simulink model "BUCK_BUCKBOOST_R2023b"  (R2023b)
settings: Solver=ode3  StartTime=0.0  StopTime=1  RelTol=1e-3
libraries: spsSeriesRLCBranchLib x56, spsCurrentMeasurementLib x42, spsVoltageMeasurementLib x27, spsMosfetLib x20, spsDiodeLib x18, spsPWMGeneratorDCDCLib x18, spsDCVoltageSourceLib x7, spsControlledVoltageSourceLib x2, spspowerguiLib x1
settings Model: Creator=tharu  LastModifiedBy=tharu
settings RTWCC: GPUComputeCapability=5.0
settings ConfigComp: CovBoundaryAbsTol=1.0e-5

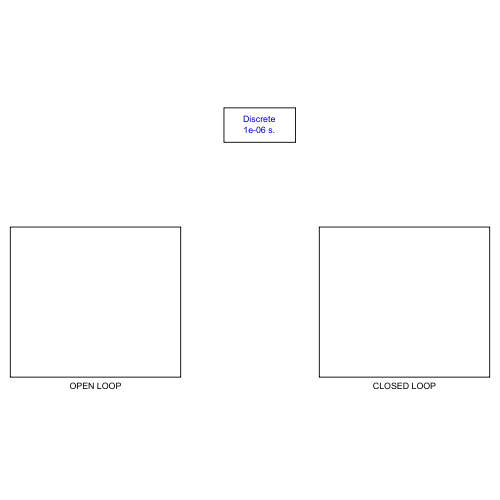
[thumbnail: Simulink's stored preview of the top-level diagram]
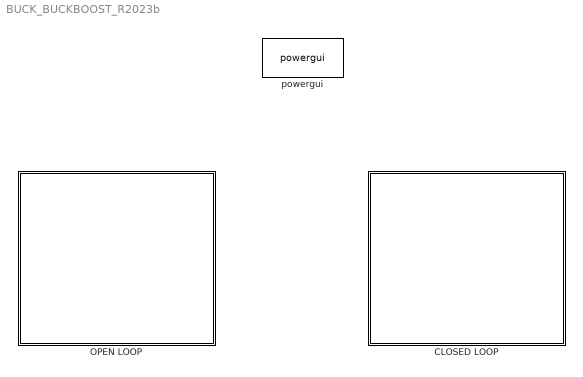
== system BUCK_BUCKBOOST_R2023b ==
  CLOSED LOOP : Subsystem
  OPEN LOOP : Subsystem
  powergui : spspowerguiLib/powergui  Priority=1  SimulationMode=Discrete  SampleTime=1e-6  frequency=60  Iterations=50  frequencyindice=0  Pbase=100e6  ErrMax=1e-4  UnitsV=kV  UnitsW=MW  buscounter=0  FunctionMessages=off  echomessages=off  EnableUseOfTLC=off  CurrentSourceSwitches=off  DisableSnubberDevices=off  DisableRonSwitches=off  DisableVfSwitches=off  DisplayEquations=off  AutomaticDiscreteSolvers=off  SolverType=Tustin/Backward Euler (TBE)  Interpol=off  ExternalGateDelay=off  methode=off  Ts=100  x0status=blocks  SPID=on  SwTol=0  HookPort=off  NonlinearTolerance=1e-4  nMaxIteration=100  ContinueOnMaxIteration=off  RestoreLinks=warning  ResistiveCurrentMeasurement=off  Frange=[0:2:500]  Ylog=off  Xlog=on  ShowGrid=off  save=off  variable=ZData  structure=0  ZoomFFT=off  StartTime=0.0  cycles=1  DisplayStyle=1  fundamental=60  FreqAxis=off  MaxFrequency=1000  frequencyindicesteady=1  RmsSteady=1  display=off

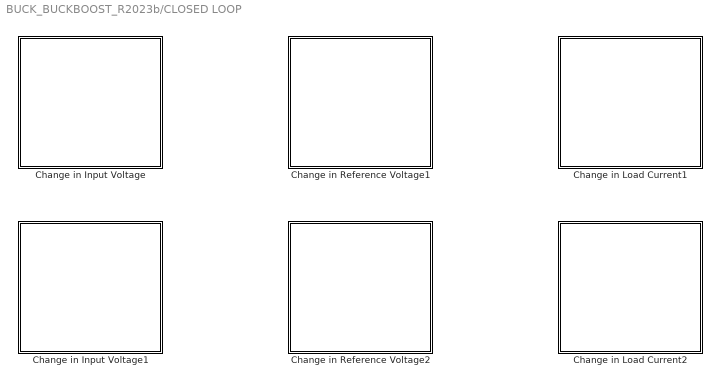
== system BUCK_BUCKBOOST_R2023b/CLOSED LOOP ==
  Change in Input Voltage : Subsystem
  Change in Input Voltage1 : Subsystem
  Change in Load Current1 : Subsystem
  Change in Load Current2 : Subsystem
  Change in Reference Voltage1 : Subsystem
  Change in Reference Voltage2 : Subsystem

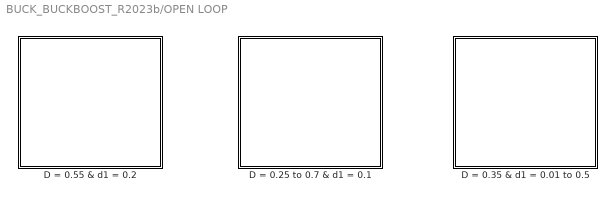
== system BUCK_BUCKBOOST_R2023b/OPEN LOOP ==
  D = 0.25 to 0.7 & d1 = 0.1 : Subsystem
  D = 0.35 & d1 = 0.01 to 0.5 : Subsystem
  D = 0.55 & d1 = 0.2 : Subsystem

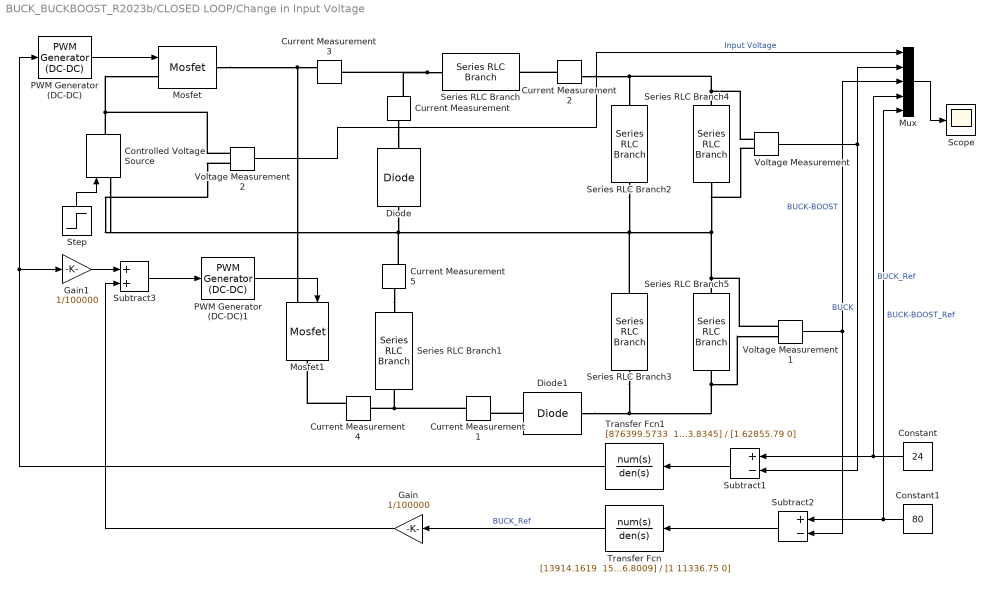
== system BUCK_BUCKBOOST_R2023b/CLOSED LOOP/Change in Input Voltage ==
  Constant : Constant  Value=24
  Constant1 : Constant  Value=80
  Controlled Voltage Source : spsControlledVoltageSourceLib/Controlled Voltage Source  Initialize=on  Source_Type=AC  Amplitude=0  Phase=0  Frequency=0  Measurements=None
  Current Measurement{,1..5} (6 alike) : spsCurrentMeasurementLib/Current Measurement  PhasorSimulation=off  OutputType=Complex  PSBequivalent=0
  Diode : spsDiodeLib/Diode  Ron=0.001  Lon=0  Vf=0.8  IC=0  UseSnubber=0  Rs=500  Cs=250e-9  Measurements=off
  Diode1 : spsDiodeLib/Diode  Ron=0.001  Lon=0  Vf=0.8  IC=0  UseSnubber=0  Rs=500  Cs=250e-9  Measurements=off
  Gain : Gain  Gain=1/100000
  Gain1 : Gain  Gain=1/100000
  Mosfet : spsMosfetLib/Mosfet  Ron=0.1  Lon=0  Rd=0.01  Vfd=0  IC=0  Rs=1e5  Cs=inf  Measurements=off
  Mosfet1 : spsMosfetLib/Mosfet  Ron=0.1  Lon=0  Rd=0.01  Vfd=0  IC=0  Rs=1e5  Cs=inf  Measurements=off
  Mux : Mux  Inputs=5
  PWM Generator (DC-DC) : spsPWMGeneratorDCDCLib/PWM Generator (DC-DC)  Fsw=50000  Ts=0
  PWM Generator (DC-DC)1 : spsPWMGeneratorDCDCLib/PWM Generator (DC-DC)  Fsw=50000  Ts=0
  Scope : Scope
  Series RLC Branch : spsSeriesRLCBranchLib/Series RLC Branch  LConnTagsString=__new0  RConnTagsString=__new0  BranchType=L  Resistance=1  Inductance=2e-3  SetiL0=off  InitialCurrent=0  Capacitance=1e-6  Setx0=off  InitialVoltage=0  Measurements=None
  Series RLC Branch1 : spsSeriesRLCBranchLib/Series RLC Branch  LConnTagsString=__new0  RConnTagsString=__new0  BranchType=L  Resistance=1  Inductance=600e-6  SetiL0=off  InitialCurrent=0  Capacitance=1e-6  Setx0=off  InitialVoltage=0  Measurements=None
  Series RLC Branch2 : spsSeriesRLCBranchLib/Series RLC Branch  LConnTagsString=__new0  RConnTagsString=__new0  BranchType=C  Resistance=1  Inductance=1e-3  SetiL0=off  InitialCurrent=0  Capacitance=100e-6  Setx0=off  InitialVoltage=0  Measurements=None
  Series RLC Branch3 : spsSeriesRLCBranchLib/Series RLC Branch  LConnTagsString=__new0  RConnTagsString=__new0  BranchType=C  Resistance=1  Inductance=1e-3  SetiL0=off  InitialCurrent=0  Capacitance=100e-6  Setx0=off  InitialVoltage=0  Measurements=None
  Series RLC Branch4 : spsSeriesRLCBranchLib/Series RLC Branch  LConnTagsString=__new0  RConnTagsString=__new0  BranchType=R  Resistance=100  Inductance=1e-3  SetiL0=off  InitialCurrent=0  Capacitance=1e-6  Setx0=off  InitialVoltage=0  Measurements=None
  Series RLC Branch5 : spsSeriesRLCBranchLib/Series RLC Branch  LConnTagsString=__new0  RConnTagsString=__new0  BranchType=R  Resistance=100  Inductance=1e-3  SetiL0=off  InitialCurrent=0  Capacitance=1e-6  Setx0=off  InitialVoltage=0  Measurements=None
  Step : Step  Time=0.5  Before=48  After=40  SampleTime=0
  Subtract1 : Sum  Inputs=+-
  Subtract2 : Sum  Inputs=+-
  Subtract3 : Sum
  Transfer Fcn : TransferFcn  Numerator="[13914.1619  15610474.6386 3044445646.8009]"  Denominator=[1 11336.75 0]
  Transfer Fcn1 : TransferFcn  Numerator="[876399.5733  1811059206.4392 399810634503.8345]"  Denominator=[1 62855.79 0]
  Voltage Measurement : spsVoltageMeasurementLib/Voltage Measurement  PhasorSimulation=off  OutputType=Complex  PSBequivalent=0
  Voltage Measurement1 : spsVoltageMeasurementLib/Voltage Measurement  PhasorSimulation=off  OutputType=Complex  PSBequivalent=0
  Voltage Measurement2 : spsVoltageMeasurementLib/Voltage Measurement  PhasorSimulation=off  OutputType=Complex  PSBequivalent=0
  wires:
  PWM Generator (DC-DC)/1 -> Mosfet/1
  Voltage Measurement1/1 -> Subtract2/2, Mux/3  "BUCK-BOOST"
  Voltage Measurement/1 -> Subtract1/2, Mux/2  "BUCK"
  Constant/1 -> Mux/4, Subtract1/1  "BUCK_Ref"
  Constant1/1 -> Subtract2/1, Mux/5  "BUCK-BOOST_Ref"
  Step/1 -> Controlled Voltage Source/1
  Mux/1 -> Scope/1
  Subtract1/1 -> Transfer Fcn1/1
  Voltage Measurement2/1 -> Mux/1  "Input Voltage"
  Subtract2/1 -> Transfer Fcn/1
  Transfer Fcn/1 -> Gain/1  "BUCK_Ref"
  Gain/1 -> Subtract3/2
  Transfer Fcn1/1 -> PWM Generator (DC-DC)/1, Gain1/1
  Gain1/1 -> Subtract3/1
  Subtract3/1 -> PWM Generator (DC-DC)1/1
  PWM Generator (DC-DC)1/1 -> Mosfet1/1
  connections:
  Diode1/LConn1 -- Series RLC Branch3/RConn1 -- Voltage Measurement1/LConn2 -- Series RLC Branch5/RConn1
  Series RLC Branch4/LConn1 -- Voltage Measurement/LConn1 -- Current Measurement2/RConn1 -- Series RLC Branch2/LConn1
  Series RLC Branch5/LConn1 -- Voltage Measurement1/LConn1 -- Voltage Measurement/LConn2 -- Series RLC Branch4/RConn1 -- Controlled Voltage Source/LConn1 -- Voltage Measurement2/LConn2 -- Current Measurement5/RConn1 -- Diode/LConn1 -- Series RLC Branch3/LConn1 -- Series RLC Branch2/RConn1
  Current Measurement1/LConn1 -- Series RLC Branch1/RConn1 -- Current Measurement4/LConn1
  Series RLC Branch/LConn1 -- Current Measurement/RConn1 -- Current Measurement3/LConn1
  Voltage Measurement2/LConn1 -- Controlled Voltage Source/RConn1 -- Mosfet/LConn1
  Diode1/RConn1 -- Current Measurement1/RConn1
  Current Measurement2/LConn1 -- Series RLC Branch/RConn1
  Current Measurement5/LConn1 -- Series RLC Branch1/LConn1
  Mosfet/RConn1 -- Mosfet1/LConn1 -- Current Measurement3/RConn1
  Current Measurement4/RConn1 -- Mosfet1/RConn1
  Current Measurement/LConn1 -- Diode/RConn1

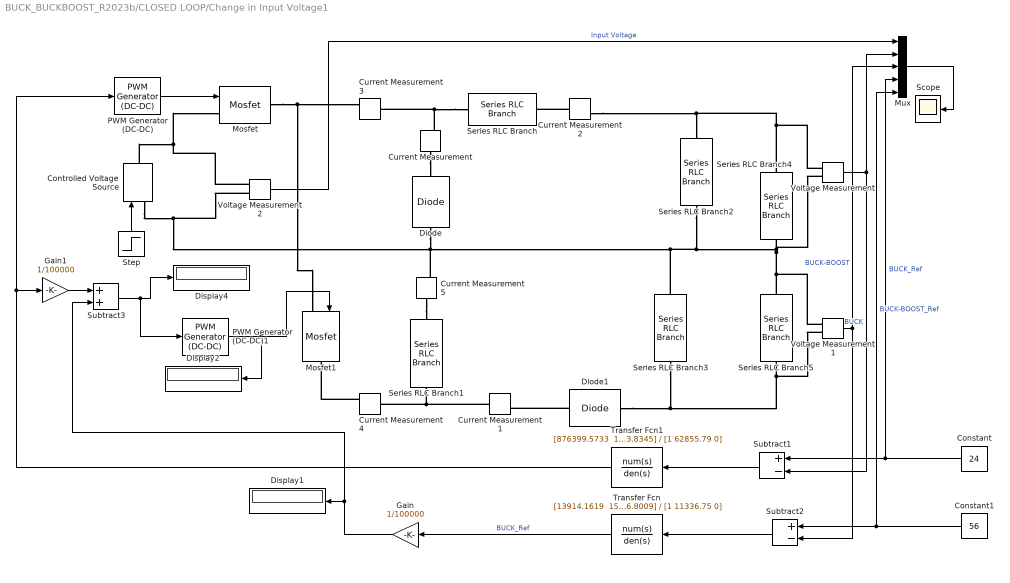
== system BUCK_BUCKBOOST_R2023b/CLOSED LOOP/Change in Input Voltage1 ==
  Constant : Constant  Value=24
  Constant1 : Constant  Value=56
  Controlled Voltage Source : spsControlledVoltageSourceLib/Controlled Voltage Source  Initialize=on  Source_Type=AC  Amplitude=0  Phase=0  Frequency=0  Measurements=None
  Current Measurement{,1..5} (6 alike) : spsCurrentMeasurementLib/Current Measurement  PhasorSimulation=off  OutputType=Complex  PSBequivalent=0
  Diode : spsDiodeLib/Diode  Ron=0.001  Lon=0  Vf=0.8  IC=0  UseSnubber=0  Rs=500  Cs=250e-9  Measurements=off
  Diode1 : spsDiodeLib/Diode  Ron=0.001  Lon=0  Vf=0.8  IC=0  UseSnubber=0  Rs=500  Cs=250e-9  Measurements=off
  Display1 : Display
  Display2 : Display
  Display4 : Display
  Gain : Gain  Gain=1/100000
  Gain1 : Gain  Gain=1/100000
  Mosfet : spsMosfetLib/Mosfet  Ron=0.1  Lon=0  Rd=0.01  Vfd=0  IC=0  Rs=1e5  Cs=inf  Measurements=off
  Mosfet1 : spsMosfetLib/Mosfet  Ron=0.1  Lon=0  Rd=0.01  Vfd=0  IC=0  Rs=1e5  Cs=inf  Measurements=off
  Mux : Mux  Inputs=5
  PWM Generator (DC-DC) : spsPWMGeneratorDCDCLib/PWM Generator (DC-DC)  Fsw=50000  Ts=0
  PWM Generator (DC-DC)1 : spsPWMGeneratorDCDCLib/PWM Generator (DC-DC)  Fsw=50000  Ts=0
  Scope : Scope
  Series RLC Branch : spsSeriesRLCBranchLib/Series RLC Branch  LConnTagsString=__new0  RConnTagsString=__new0  BranchType=L  Resistance=1  Inductance=2e-3  SetiL0=off  InitialCurrent=0  Capacitance=1e-6  Setx0=off  InitialVoltage=0  Measurements=None
  Series RLC Branch1 : spsSeriesRLCBranchLib/Series RLC Branch  LConnTagsString=__new0  RConnTagsString=__new0  BranchType=L  Resistance=1  Inductance=600e-6  SetiL0=off  InitialCurrent=0  Capacitance=1e-6  Setx0=off  InitialVoltage=0  Measurements=None
  Series RLC Branch2 : spsSeriesRLCBranchLib/Series RLC Branch  LConnTagsString=__new0  RConnTagsString=__new0  BranchType=C  Resistance=1  Inductance=1e-3  SetiL0=off  InitialCurrent=0  Capacitance=100e-6  Setx0=off  InitialVoltage=0  Measurements=None
  Series RLC Branch3 : spsSeriesRLCBranchLib/Series RLC Branch  LConnTagsString=__new0  RConnTagsString=__new0  BranchType=C  Resistance=1  Inductance=1e-3  SetiL0=off  InitialCurrent=0  Capacitance=100e-6  Setx0=off  InitialVoltage=0  Measurements=None
  Series RLC Branch4 : spsSeriesRLCBranchLib/Series RLC Branch  LConnTagsString=__new0  RConnTagsString=__new0  BranchType=R  Resistance=100  Inductance=1e-3  SetiL0=off  InitialCurrent=0  Capacitance=1e-6  Setx0=off  InitialVoltage=0  Measurements=None
  Series RLC Branch5 : spsSeriesRLCBranchLib/Series RLC Branch  LConnTagsString=__new0  RConnTagsString=__new0  BranchType=R  Resistance=100  Inductance=1e-3  SetiL0=off  InitialCurrent=0  Capacitance=1e-6  Setx0=off  InitialVoltage=0  Measurements=None
  Step : Step  Time=0.5  Before=48  After=40  SampleTime=0
  Subtract1 : Sum  Inputs=+-
  Subtract2 : Sum  Inputs=+-
  Subtract3 : Sum
  Transfer Fcn : TransferFcn  Numerator="[13914.1619  15610474.6386 3044445646.8009]"  Denominator=[1 11336.75 0]
  Transfer Fcn1 : TransferFcn  Numerator="[876399.5733  1811059206.4392 399810634503.8345]"  Denominator=[1 62855.79 0]
  Voltage Measurement : spsVoltageMeasurementLib/Voltage Measurement  PhasorSimulation=off  OutputType=Complex  PSBequivalent=0
  Voltage Measurement1 : spsVoltageMeasurementLib/Voltage Measurement  PhasorSimulation=off  OutputType=Complex  PSBequivalent=0
  Voltage Measurement2 : spsVoltageMeasurementLib/Voltage Measurement  PhasorSimulation=off  OutputType=Complex  PSBequivalent=0
  wires:
  PWM Generator (DC-DC)/1 -> Mosfet/1
  Voltage Measurement1/1 -> Subtract2/2, Mux/3  "BUCK-BOOST"
  Voltage Measurement/1 -> Subtract1/2, Mux/2  "BUCK"
  Constant/1 -> Mux/4, Subtract1/1  "BUCK_Ref"
  Constant1/1 -> Mux/5, Subtract2/1  "BUCK-BOOST_Ref"
  Step/1 -> Controlled Voltage Source/1
  Mux/1 -> Scope/1
  Subtract1/1 -> Transfer Fcn1/1
  Voltage Measurement2/1 -> Mux/1  "Input Voltage"
  Subtract2/1 -> Transfer Fcn/1
  PWM Generator (DC-DC)1/1 -> Display2/1, Mosfet1/1
  Transfer Fcn/1 -> Gain/1  "BUCK_Ref"
  Gain/1 -> Subtract3/2, Display1/1
  Transfer Fcn1/1 -> Gain1/1, PWM Generator (DC-DC)/1
  Gain1/1 -> Subtract3/1
  Subtract3/1 -> PWM Generator (DC-DC)1/1, Display4/1
  connections:
  Diode1/LConn1 -- Series RLC Branch3/RConn1 -- Voltage Measurement1/LConn2 -- Series RLC Branch5/RConn1
  Series RLC Branch4/LConn1 -- Voltage Measurement/LConn1 -- Current Measurement2/RConn1 -- Series RLC Branch2/LConn1
  Series RLC Branch5/LConn1 -- Voltage Measurement1/LConn1 -- Controlled Voltage Source/LConn1 -- Voltage Measurement2/LConn2 -- Current Measurement5/RConn1 -- Diode/LConn1 -- Series RLC Branch3/LConn1 -- Series RLC Branch2/RConn1 -- Voltage Measurement/LConn2 -- Series RLC Branch4/RConn1
  Current Measurement1/LConn1 -- Series RLC Branch1/RConn1 -- Current Measurement4/LConn1
  Series RLC Branch/LConn1 -- Current Measurement/RConn1 -- Current Measurement3/LConn1
  Voltage Measurement2/LConn1 -- Controlled Voltage Source/RConn1 -- Mosfet/LConn1
  Diode1/RConn1 -- Current Measurement1/RConn1
  Current Measurement2/LConn1 -- Series RLC Branch/RConn1
  Current Measurement5/LConn1 -- Series RLC Branch1/LConn1
  Mosfet/RConn1 -- Mosfet1/LConn1 -- Current Measurement3/RConn1
  Current Measurement4/RConn1 -- Mosfet1/RConn1
  Current Measurement/LConn1 -- Diode/RConn1

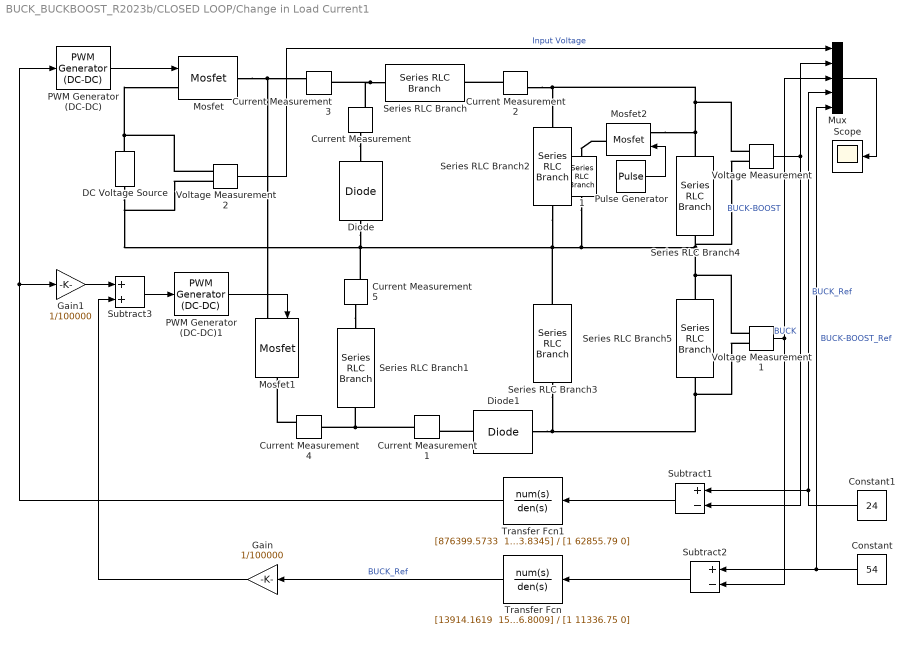
== system BUCK_BUCKBOOST_R2023b/CLOSED LOOP/Change in Load Current1 ==
  1 : spsSeriesRLCBranchLib/Series RLC Branch  LConnTagsString=__new0  RConnTagsString=__new0  BranchType=R  Resistance=22  Inductance=1e-3  SetiL0=off  InitialCurrent=0  Capacitance=1e-6  Setx0=off  InitialVoltage=0  Measurements=None
  Constant : Constant  Value=54
  Constant1 : Constant  Value=24
  Current Measurement{,1..5} (6 alike) : spsCurrentMeasurementLib/Current Measurement  PhasorSimulation=off  OutputType=Complex  PSBequivalent=0
  DC Voltage Source : spsDCVoltageSourceLib/DC Voltage Source  Amplitude=48  Measurements=None
  Diode : spsDiodeLib/Diode  Ron=0.001  Lon=0  Vf=0.8  IC=0  UseSnubber=0  Rs=500  Cs=250e-9  Measurements=off
  Diode1 : spsDiodeLib/Diode  Ron=0.001  Lon=0  Vf=0.8  IC=0  UseSnubber=0  Rs=500  Cs=250e-9  Measurements=off
  Gain : Gain  Gain=1/100000
  Gain1 : Gain  Gain=1/100000
  Mosfet : spsMosfetLib/Mosfet  Ron=0.1  Lon=0  Rd=0.01  Vfd=0  IC=0  Rs=1e5  Cs=inf  Measurements=off
  Mosfet1 : spsMosfetLib/Mosfet  Ron=0.1  Lon=0  Rd=0.01  Vfd=0  IC=0  Rs=1e5  Cs=inf  Measurements=off
  Mosfet2 : spsMosfetLib/Mosfet  Ron=0.1  Lon=0  Rd=0.01  Vfd=0  IC=0  Rs=1e5  Cs=inf  Measurements=off
  Mux : Mux  Inputs=5
  PWM Generator (DC-DC) : spsPWMGeneratorDCDCLib/PWM Generator (DC-DC)  Fsw=50000  Ts=0
  PWM Generator (DC-DC)1 : spsPWMGeneratorDCDCLib/PWM Generator (DC-DC)  Fsw=50000  Ts=0
  Pulse Generator : DiscretePulseGenerator  PulseType=Time based  Period=.1  PulseWidth=40  PhaseDelay=0.040
  Scope : Scope
  Series RLC Branch : spsSeriesRLCBranchLib/Series RLC Branch  LConnTagsString=__new0  RConnTagsString=__new0  BranchType=L  Resistance=1  Inductance=2e-3  SetiL0=off  InitialCurrent=0  Capacitance=1e-6  Setx0=off  InitialVoltage=0  Measurements=None
  Series RLC Branch1 : spsSeriesRLCBranchLib/Series RLC Branch  LConnTagsString=__new0  RConnTagsString=__new0  BranchType=L  Resistance=1  Inductance=600e-6  SetiL0=off  InitialCurrent=0  Capacitance=1e-6  Setx0=off  InitialVoltage=0  Measurements=None
  Series RLC Branch2 : spsSeriesRLCBranchLib/Series RLC Branch  LConnTagsString=__new0  RConnTagsString=__new0  BranchType=C  Resistance=1  Inductance=1e-3  SetiL0=off  InitialCurrent=0  Capacitance=100e-6  Setx0=off  InitialVoltage=0  Measurements=None
  Series RLC Branch3 : spsSeriesRLCBranchLib/Series RLC Branch  LConnTagsString=__new0  RConnTagsString=__new0  BranchType=C  Resistance=1  Inductance=1e-3  SetiL0=off  InitialCurrent=0  Capacitance=100e-6  Setx0=off  InitialVoltage=0  Measurements=None
  Series RLC Branch4 : spsSeriesRLCBranchLib/Series RLC Branch  LConnTagsString=__new0  RConnTagsString=__new0  BranchType=R  Resistance=100  Inductance=1e-3  SetiL0=off  InitialCurrent=0  Capacitance=1e-6  Setx0=off  InitialVoltage=0  Measurements=None
  Series RLC Branch5 : spsSeriesRLCBranchLib/Series RLC Branch  LConnTagsString=__new0  RConnTagsString=__new0  BranchType=R  Resistance=100  Inductance=1e-3  SetiL0=off  InitialCurrent=0  Capacitance=1e-6  Setx0=off  InitialVoltage=0  Measurements=None
  Subtract1 : Sum  Inputs=+-
  Subtract2 : Sum  Inputs=+-
  Subtract3 : Sum
  Transfer Fcn : TransferFcn  Numerator="[13914.1619  15610474.6386 3044445646.8009]"  Denominator=[1 11336.75 0]
  Transfer Fcn1 : TransferFcn  Numerator="[876399.5733  1811059206.4392 399810634503.8345]"  Denominator=[1 62855.79 0]
  Voltage Measurement : spsVoltageMeasurementLib/Voltage Measurement  PhasorSimulation=off  OutputType=Complex  PSBequivalent=0
  Voltage Measurement1 : spsVoltageMeasurementLib/Voltage Measurement  PhasorSimulation=off  OutputType=Complex  PSBequivalent=0
  Voltage Measurement2 : spsVoltageMeasurementLib/Voltage Measurement  PhasorSimulation=off  OutputType=Complex  PSBequivalent=0
  wires:
  PWM Generator (DC-DC)/1 -> Mosfet/1
  Voltage Measurement1/1 -> Subtract2/2, Mux/3  "BUCK-BOOST"
  Voltage Measurement/1 -> Subtract1/2, Mux/2  "BUCK"
  Constant1/1 -> Mux/4, Subtract1/1  "BUCK_Ref"
  Constant/1 -> Mux/5, Subtract2/1  "BUCK-BOOST_Ref"
  Mux/1 -> Scope/1
  Subtract1/1 -> Transfer Fcn1/1
  Voltage Measurement2/1 -> Mux/1  "Input Voltage"
  Subtract2/1 -> Transfer Fcn/1
  PWM Generator (DC-DC)1/1 -> Mosfet1/1
  Transfer Fcn/1 -> Gain/1  "BUCK_Ref"
  Gain/1 -> Subtract3/2
  Transfer Fcn1/1 -> PWM Generator (DC-DC)/1, Gain1/1
  Gain1/1 -> Subtract3/1
  Subtract3/1 -> PWM Generator (DC-DC)1/1
  Pulse Generator/1 -> Mosfet2/1
  connections:
  Diode1/LConn1 -- Voltage Measurement1/LConn2 -- Series RLC Branch5/RConn1 -- Series RLC Branch3/RConn1
  Series RLC Branch4/LConn1 -- Mosfet2/LConn1 -- Voltage Measurement/LConn1 -- Current Measurement2/RConn1 -- Series RLC Branch2/LConn1
  Series RLC Branch5/LConn1 -- Voltage Measurement1/LConn1 -- Series RLC Branch4/RConn1 -- Voltage Measurement2/LConn2 -- DC Voltage Source/LConn1 -- Current Measurement5/RConn1 -- Diode/LConn1 -- Series RLC Branch2/RConn1 -- Series RLC Branch3/LConn1 -- 1/RConn1 -- Voltage Measurement/LConn2
  Current Measurement1/LConn1 -- Current Measurement4/LConn1 -- Series RLC Branch1/RConn1
  Series RLC Branch/LConn1 -- Current Measurement3/LConn1 -- Current Measurement/RConn1
  DC Voltage Source/RConn1 -- Voltage Measurement2/LConn1 -- Mosfet/LConn1
  Diode1/RConn1 -- Current Measurement1/RConn1
  Current Measurement2/LConn1 -- Series RLC Branch/RConn1
  Current Measurement5/LConn1 -- Series RLC Branch1/LConn1
  Mosfet/RConn1 -- Mosfet1/LConn1 -- Current Measurement3/RConn1
  Current Measurement4/RConn1 -- Mosfet1/RConn1
  Current Measurement/LConn1 -- Diode/RConn1
  Mosfet2/RConn1 -- 1/LConn1

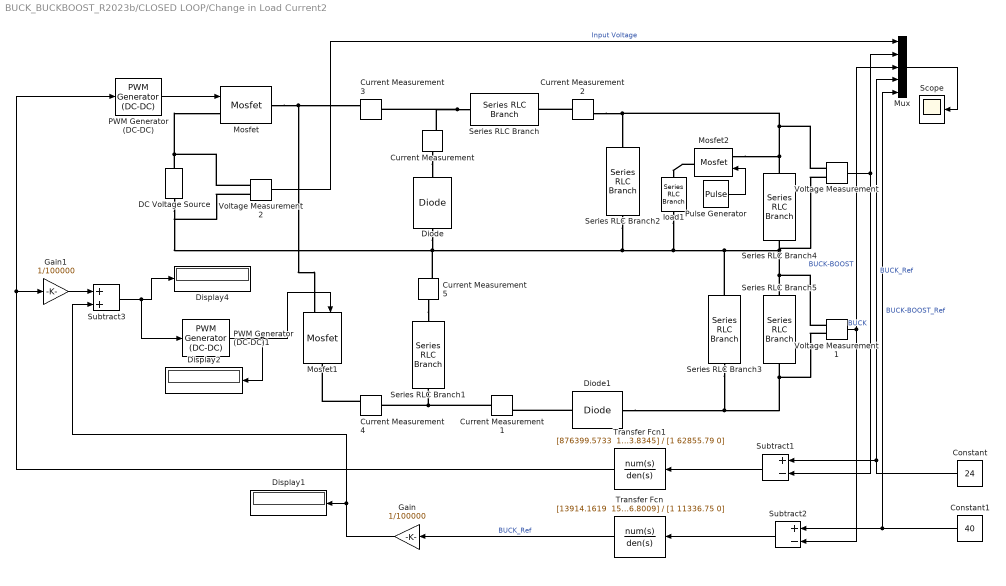
== system BUCK_BUCKBOOST_R2023b/CLOSED LOOP/Change in Load Current2 ==
  Constant : Constant  Value=24
  Constant1 : Constant  Value=40
  Current Measurement{,1..5} (6 alike) : spsCurrentMeasurementLib/Current Measurement  PhasorSimulation=off  OutputType=Complex  PSBequivalent=0
  DC Voltage Source : spsDCVoltageSourceLib/DC Voltage Source  Amplitude=48  Measurements=None
  Diode : spsDiodeLib/Diode  Ron=0.001  Lon=0  Vf=0.8  IC=0  UseSnubber=0  Rs=500  Cs=250e-9  Measurements=off
  Diode1 : spsDiodeLib/Diode  Ron=0.001  Lon=0  Vf=0.8  IC=0  UseSnubber=0  Rs=500  Cs=250e-9  Measurements=off
  Display1 : Display
  Display2 : Display
  Display4 : Display
  Gain : Gain  Gain=1/100000
  Gain1 : Gain  Gain=1/100000
  Mosfet : spsMosfetLib/Mosfet  Ron=0.1  Lon=0  Rd=0.01  Vfd=0  IC=0  Rs=1e5  Cs=inf  Measurements=off
  Mosfet1 : spsMosfetLib/Mosfet  Ron=0.1  Lon=0  Rd=0.01  Vfd=0  IC=0  Rs=1e5  Cs=inf  Measurements=off
  Mosfet2 : spsMosfetLib/Mosfet  Ron=0.1  Lon=0  Rd=0.01  Vfd=0  IC=0  Rs=1e5  Cs=inf  Measurements=off
  Mux : Mux  Inputs=5
  PWM Generator (DC-DC) : spsPWMGeneratorDCDCLib/PWM Generator (DC-DC)  Fsw=50000  Ts=0
  PWM Generator (DC-DC)1 : spsPWMGeneratorDCDCLib/PWM Generator (DC-DC)  Fsw=50000  Ts=0
  Pulse Generator : DiscretePulseGenerator  PulseType=Time based  Period=.1  PulseWidth=40  PhaseDelay=0.040
  Scope : Scope
  Series RLC Branch : spsSeriesRLCBranchLib/Series RLC Branch  LConnTagsString=__new0  RConnTagsString=__new0  BranchType=L  Resistance=1  Inductance=2e-3  SetiL0=off  InitialCurrent=0  Capacitance=1e-6  Setx0=off  InitialVoltage=0  Measurements=None
  Series RLC Branch1 : spsSeriesRLCBranchLib/Series RLC Branch  LConnTagsString=__new0  RConnTagsString=__new0  BranchType=L  Resistance=1  Inductance=600e-6  SetiL0=off  InitialCurrent=0  Capacitance=1e-6  Setx0=off  InitialVoltage=0  Measurements=None
  Series RLC Branch2 : spsSeriesRLCBranchLib/Series RLC Branch  LConnTagsString=__new0  RConnTagsString=__new0  BranchType=C  Resistance=1  Inductance=1e-3  SetiL0=off  InitialCurrent=0  Capacitance=100e-6  Setx0=off  InitialVoltage=0  Measurements=None
  Series RLC Branch3 : spsSeriesRLCBranchLib/Series RLC Branch  LConnTagsString=__new0  RConnTagsString=__new0  BranchType=C  Resistance=1  Inductance=1e-3  SetiL0=off  InitialCurrent=0  Capacitance=100e-6  Setx0=off  InitialVoltage=0  Measurements=None
  Series RLC Branch4 : spsSeriesRLCBranchLib/Series RLC Branch  LConnTagsString=__new0  RConnTagsString=__new0  BranchType=R  Resistance=100  Inductance=1e-3  SetiL0=off  InitialCurrent=0  Capacitance=1e-6  Setx0=off  InitialVoltage=0  Measurements=None
  Series RLC Branch5 : spsSeriesRLCBranchLib/Series RLC Branch  LConnTagsString=__new0  RConnTagsString=__new0  BranchType=R  Resistance=100  Inductance=1e-3  SetiL0=off  InitialCurrent=0  Capacitance=1e-6  Setx0=off  InitialVoltage=0  Measurements=None
  Subtract1 : Sum  Inputs=+-
  Subtract2 : Sum  Inputs=+-
  Subtract3 : Sum
  Transfer Fcn : TransferFcn  Numerator="[13914.1619  15610474.6386 3044445646.8009]"  Denominator=[1 11336.75 0]
  Transfer Fcn1 : TransferFcn  Numerator="[876399.5733  1811059206.4392 399810634503.8345]"  Denominator=[1 62855.79 0]
  Voltage Measurement : spsVoltageMeasurementLib/Voltage Measurement  PhasorSimulation=off  OutputType=Complex  PSBequivalent=0
  Voltage Measurement1 : spsVoltageMeasurementLib/Voltage Measurement  PhasorSimulation=off  OutputType=Complex  PSBequivalent=0
  Voltage Measurement2 : spsVoltageMeasurementLib/Voltage Measurement  PhasorSimulation=off  OutputType=Complex  PSBequivalent=0
  load1 : spsSeriesRLCBranchLib/Series RLC Branch  LConnTagsString=__new0  RConnTagsString=__new0  BranchType=R  Resistance=22  Inductance=1e-3  SetiL0=off  InitialCurrent=0  Capacitance=1e-6  Setx0=off  InitialVoltage=0  Measurements=None
  wires:
  PWM Generator (DC-DC)/1 -> Mosfet/1
  Voltage Measurement1/1 -> Subtract2/2, Mux/3  "BUCK-BOOST"
  Voltage Measurement/1 -> Subtract1/2, Mux/2  "BUCK"
  Constant/1 -> Mux/4, Subtract1/1  "BUCK_Ref"
  Constant1/1 -> Subtract2/1, Mux/5  "BUCK-BOOST_Ref"
  Mux/1 -> Scope/1
  Subtract1/1 -> Transfer Fcn1/1
  Voltage Measurement2/1 -> Mux/1  "Input Voltage"
  Subtract2/1 -> Transfer Fcn/1
  PWM Generator (DC-DC)1/1 -> Display2/1, Mosfet1/1
  Transfer Fcn/1 -> Gain/1  "BUCK_Ref"
  Gain/1 -> Subtract3/2, Display1/1
  Transfer Fcn1/1 -> Gain1/1, PWM Generator (DC-DC)/1
  Gain1/1 -> Subtract3/1
  Subtract3/1 -> PWM Generator (DC-DC)1/1, Display4/1
  Pulse Generator/1 -> Mosfet2/1
  connections:
  Diode1/LConn1 -- Series RLC Branch3/RConn1 -- Voltage Measurement1/LConn2 -- Series RLC Branch5/RConn1
  Series RLC Branch4/LConn1 -- Voltage Measurement/LConn1 -- Current Measurement2/RConn1 -- Series RLC Branch2/LConn1 -- Mosfet2/LConn1
  Series RLC Branch5/LConn1 -- Voltage Measurement1/LConn1 -- Series RLC Branch4/RConn1 -- load1/RConn1 -- Series RLC Branch2/RConn1 -- Current Measurement5/RConn1 -- Diode/LConn1 -- Voltage Measurement2/LConn2 -- DC Voltage Source/LConn1 -- Series RLC Branch3/LConn1 -- Voltage Measurement/LConn2
  Current Measurement1/LConn1 -- Series RLC Branch1/RConn1 -- Current Measurement4/LConn1
  Series RLC Branch/LConn1 -- Current Measurement/RConn1 -- Current Measurement3/LConn1
  DC Voltage Source/RConn1 -- Voltage Measurement2/LConn1 -- Mosfet/LConn1
  Diode1/RConn1 -- Current Measurement1/RConn1
  Current Measurement2/LConn1 -- Series RLC Branch/RConn1
  Current Measurement5/LConn1 -- Series RLC Branch1/LConn1
  Mosfet/RConn1 -- Mosfet1/LConn1 -- Current Measurement3/RConn1
  Current Measurement4/RConn1 -- Mosfet1/RConn1
  Current Measurement/LConn1 -- Diode/RConn1
  Mosfet2/RConn1 -- load1/LConn1

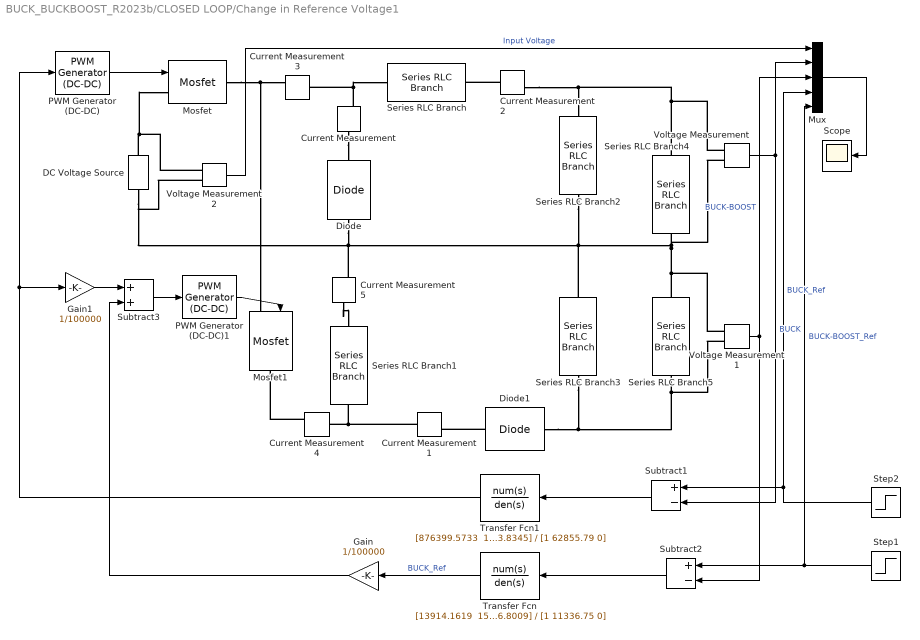
== system BUCK_BUCKBOOST_R2023b/CLOSED LOOP/Change in Reference Voltage1 ==
  Current Measurement{,1..5} (6 alike) : spsCurrentMeasurementLib/Current Measurement  PhasorSimulation=off  OutputType=Complex  PSBequivalent=0
  DC Voltage Source : spsDCVoltageSourceLib/DC Voltage Source  Amplitude=48  Measurements=None
  Diode : spsDiodeLib/Diode  Ron=0.001  Lon=0  Vf=0.8  IC=0  UseSnubber=0  Rs=500  Cs=250e-9  Measurements=off
  Diode1 : spsDiodeLib/Diode  Ron=0.001  Lon=0  Vf=0.8  IC=0  UseSnubber=0  Rs=500  Cs=250e-9  Measurements=off
  Gain : Gain  Gain=1/100000
  Gain1 : Gain  Gain=1/100000
  Mosfet : spsMosfetLib/Mosfet  Ron=0.1  Lon=0  Rd=0.01  Vfd=0  IC=0  Rs=1e5  Cs=inf  Measurements=off
  Mosfet1 : spsMosfetLib/Mosfet  Ron=0.1  Lon=0  Rd=0.01  Vfd=0  IC=0  Rs=1e5  Cs=inf  Measurements=off
  Mux : Mux  Inputs=5
  PWM Generator (DC-DC) : spsPWMGeneratorDCDCLib/PWM Generator (DC-DC)  Fsw=50000  Ts=0
  PWM Generator (DC-DC)1 : spsPWMGeneratorDCDCLib/PWM Generator (DC-DC)  Fsw=50000  Ts=0
  Scope : Scope
  Series RLC Branch : spsSeriesRLCBranchLib/Series RLC Branch  LConnTagsString=__new0  RConnTagsString=__new0  BranchType=L  Resistance=1  Inductance=2e-3  SetiL0=off  InitialCurrent=0  Capacitance=1e-6  Setx0=off  InitialVoltage=0  Measurements=None
  Series RLC Branch1 : spsSeriesRLCBranchLib/Series RLC Branch  LConnTagsString=__new0  RConnTagsString=__new0  BranchType=L  Resistance=1  Inductance=600e-6  SetiL0=off  InitialCurrent=0  Capacitance=1e-6  Setx0=off  InitialVoltage=0  Measurements=None
  Series RLC Branch2 : spsSeriesRLCBranchLib/Series RLC Branch  LConnTagsString=__new0  RConnTagsString=__new0  BranchType=C  Resistance=1  Inductance=1e-3  SetiL0=off  InitialCurrent=0  Capacitance=100e-6  Setx0=off  InitialVoltage=0  Measurements=None
  Series RLC Branch3 : spsSeriesRLCBranchLib/Series RLC Branch  LConnTagsString=__new0  RConnTagsString=__new0  BranchType=C  Resistance=1  Inductance=1e-3  SetiL0=off  InitialCurrent=0  Capacitance=100e-6  Setx0=off  InitialVoltage=0  Measurements=None
  Series RLC Branch4 : spsSeriesRLCBranchLib/Series RLC Branch  LConnTagsString=__new0  RConnTagsString=__new0  BranchType=R  Resistance=100  Inductance=1e-3  SetiL0=off  InitialCurrent=0  Capacitance=1e-6  Setx0=off  InitialVoltage=0  Measurements=None
  Series RLC Branch5 : spsSeriesRLCBranchLib/Series RLC Branch  LConnTagsString=__new0  RConnTagsString=__new0  BranchType=R  Resistance=100  Inductance=1e-3  SetiL0=off  InitialCurrent=0  Capacitance=1e-6  Setx0=off  InitialVoltage=0  Measurements=None
  Step1 : Step  Time=0.5  Before=80  After=54  SampleTime=0
  Step2 : Step  Time=0.5  Before=24  After=36  SampleTime=0
  Subtract1 : Sum  Inputs=+-
  Subtract2 : Sum  Inputs=+-
  Subtract3 : Sum
  Transfer Fcn : TransferFcn  Numerator="[13914.1619  15610474.6386 3044445646.8009]"  Denominator=[1 11336.75 0]
  Transfer Fcn1 : TransferFcn  Numerator="[876399.5733  1811059206.4392 399810634503.8345]"  Denominator=[1 62855.79 0]
  Voltage Measurement : spsVoltageMeasurementLib/Voltage Measurement  PhasorSimulation=off  OutputType=Complex  PSBequivalent=0
  Voltage Measurement1 : spsVoltageMeasurementLib/Voltage Measurement  PhasorSimulation=off  OutputType=Complex  PSBequivalent=0
  Voltage Measurement2 : spsVoltageMeasurementLib/Voltage Measurement  PhasorSimulation=off  OutputType=Complex  PSBequivalent=0
  wires:
  PWM Generator (DC-DC)/1 -> Mosfet/1
  Voltage Measurement1/1 -> Subtract2/2, Mux/3  "BUCK-BOOST"
  Voltage Measurement/1 -> Subtract1/2, Mux/2  "BUCK"
  Step2/1 -> Mux/4, Subtract1/1  "BUCK_Ref"
  Step1/1 -> Mux/5, Subtract2/1  "BUCK-BOOST_Ref"
  Mux/1 -> Scope/1
  Subtract1/1 -> Transfer Fcn1/1
  Voltage Measurement2/1 -> Mux/1  "Input Voltage"
  Subtract2/1 -> Transfer Fcn/1
  PWM Generator (DC-DC)1/1 -> Mosfet1/1
  Transfer Fcn/1 -> Gain/1  "BUCK_Ref"
  Gain/1 -> Subtract3/2
  Transfer Fcn1/1 -> Gain1/1, PWM Generator (DC-DC)/1
  Gain1/1 -> Subtract3/1
  Subtract3/1 -> PWM Generator (DC-DC)1/1
  connections:
  Diode1/LConn1 -- Voltage Measurement1/LConn2 -- Series RLC Branch5/RConn1 -- Series RLC Branch3/RConn1
  Series RLC Branch4/LConn1 -- Voltage Measurement/LConn1 -- Current Measurement2/RConn1 -- Series RLC Branch2/LConn1
  Series RLC Branch5/LConn1 -- Voltage Measurement1/LConn1 -- Series RLC Branch4/RConn1 -- Voltage Measurement/LConn2 -- Voltage Measurement2/LConn2 -- DC Voltage Source/LConn1 -- Current Measurement5/RConn1 -- Diode/LConn1 -- Series RLC Branch3/LConn1 -- Series RLC Branch2/RConn1
  Current Measurement1/LConn1 -- Series RLC Branch1/RConn1 -- Current Measurement4/LConn1
  Current Measurement/RConn1 -- Series RLC Branch/LConn1 -- Current Measurement3/LConn1
  DC Voltage Source/RConn1 -- Voltage Measurement2/LConn1 -- Mosfet/LConn1
  Diode1/RConn1 -- Current Measurement1/RConn1
  Current Measurement2/LConn1 -- Series RLC Branch/RConn1
  Current Measurement5/LConn1 -- Series RLC Branch1/LConn1
  Mosfet/RConn1 -- Current Measurement3/RConn1 -- Mosfet1/LConn1
  Current Measurement4/RConn1 -- Mosfet1/RConn1
  Current Measurement/LConn1 -- Diode/RConn1

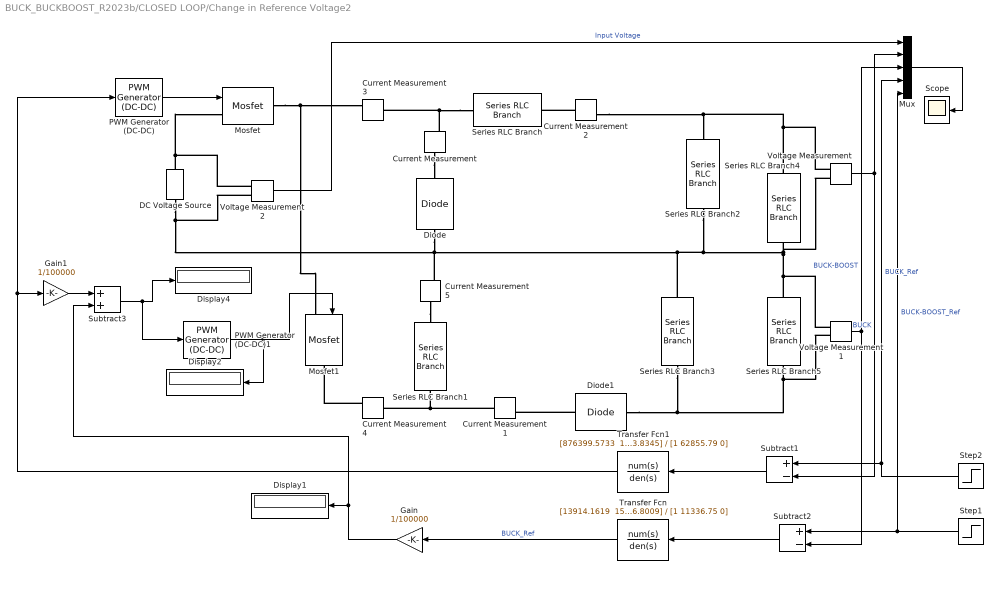
== system BUCK_BUCKBOOST_R2023b/CLOSED LOOP/Change in Reference Voltage2 ==
  Current Measurement{,1..5} (6 alike) : spsCurrentMeasurementLib/Current Measurement  PhasorSimulation=off  OutputType=Complex  PSBequivalent=0
  DC Voltage Source : spsDCVoltageSourceLib/DC Voltage Source  Amplitude=48  Measurements=None
  Diode : spsDiodeLib/Diode  Ron=0.001  Lon=0  Vf=0.8  IC=0  UseSnubber=0  Rs=500  Cs=250e-9  Measurements=off
  Diode1 : spsDiodeLib/Diode  Ron=0.001  Lon=0  Vf=0.8  IC=0  UseSnubber=0  Rs=500  Cs=250e-9  Measurements=off
  Display1 : Display
  Display2 : Display
  Display4 : Display
  Gain : Gain  Gain=1/100000
  Gain1 : Gain  Gain=1/100000
  Mosfet : spsMosfetLib/Mosfet  Ron=0.1  Lon=0  Rd=0.01  Vfd=0  IC=0  Rs=1e5  Cs=inf  Measurements=off
  Mosfet1 : spsMosfetLib/Mosfet  Ron=0.1  Lon=0  Rd=0.01  Vfd=0  IC=0  Rs=1e5  Cs=inf  Measurements=off
  Mux : Mux  Inputs=5
  PWM Generator (DC-DC) : spsPWMGeneratorDCDCLib/PWM Generator (DC-DC)  Fsw=50000  Ts=0
  PWM Generator (DC-DC)1 : spsPWMGeneratorDCDCLib/PWM Generator (DC-DC)  Fsw=50000  Ts=0
  Scope : Scope
  Series RLC Branch : spsSeriesRLCBranchLib/Series RLC Branch  LConnTagsString=__new0  RConnTagsString=__new0  BranchType=L  Resistance=1  Inductance=2e-3  SetiL0=off  InitialCurrent=0  Capacitance=1e-6  Setx0=off  InitialVoltage=0  Measurements=None
  Series RLC Branch1 : spsSeriesRLCBranchLib/Series RLC Branch  LConnTagsString=__new0  RConnTagsString=__new0  BranchType=L  Resistance=1  Inductance=600e-6  SetiL0=off  InitialCurrent=0  Capacitance=1e-6  Setx0=off  InitialVoltage=0  Measurements=None
  Series RLC Branch2 : spsSeriesRLCBranchLib/Series RLC Branch  LConnTagsString=__new0  RConnTagsString=__new0  BranchType=C  Resistance=1  Inductance=1e-3  SetiL0=off  InitialCurrent=0  Capacitance=100e-6  Setx0=off  InitialVoltage=0  Measurements=None
  Series RLC Branch3 : spsSeriesRLCBranchLib/Series RLC Branch  LConnTagsString=__new0  RConnTagsString=__new0  BranchType=C  Resistance=1  Inductance=1e-3  SetiL0=off  InitialCurrent=0  Capacitance=100e-6  Setx0=off  InitialVoltage=0  Measurements=None
  Series RLC Branch4 : spsSeriesRLCBranchLib/Series RLC Branch  LConnTagsString=__new0  RConnTagsString=__new0  BranchType=R  Resistance=100  Inductance=1e-3  SetiL0=off  InitialCurrent=0  Capacitance=1e-6  Setx0=off  InitialVoltage=0  Measurements=None
  Series RLC Branch5 : spsSeriesRLCBranchLib/Series RLC Branch  LConnTagsString=__new0  RConnTagsString=__new0  BranchType=R  Resistance=100  Inductance=1e-3  SetiL0=off  InitialCurrent=0  Capacitance=1e-6  Setx0=off  InitialVoltage=0  Measurements=None
  Step1 : Step  Time=0.5  Before=30  After=40  SampleTime=0
  Step2 : Step  Time=0.5  Before=24  After=36  SampleTime=0
  Subtract1 : Sum  Inputs=+-
  Subtract2 : Sum  Inputs=+-
  Subtract3 : Sum
  Transfer Fcn : TransferFcn  Numerator="[13914.1619  15610474.6386 3044445646.8009]"  Denominator=[1 11336.75 0]
  Transfer Fcn1 : TransferFcn  Numerator="[876399.5733  1811059206.4392 399810634503.8345]"  Denominator=[1 62855.79 0]
  Voltage Measurement : spsVoltageMeasurementLib/Voltage Measurement  PhasorSimulation=off  OutputType=Complex  PSBequivalent=0
  Voltage Measurement1 : spsVoltageMeasurementLib/Voltage Measurement  PhasorSimulation=off  OutputType=Complex  PSBequivalent=0
  Voltage Measurement2 : spsVoltageMeasurementLib/Voltage Measurement  PhasorSimulation=off  OutputType=Complex  PSBequivalent=0
  wires:
  PWM Generator (DC-DC)/1 -> Mosfet/1
  Voltage Measurement1/1 -> Subtract2/2, Mux/3  "BUCK-BOOST"
  Voltage Measurement/1 -> Subtract1/2, Mux/2  "BUCK"
  Step2/1 -> Mux/4, Subtract1/1  "BUCK_Ref"
  Step1/1 -> Mux/5, Subtract2/1  "BUCK-BOOST_Ref"
  Mux/1 -> Scope/1
  Subtract1/1 -> Transfer Fcn1/1
  Voltage Measurement2/1 -> Mux/1  "Input Voltage"
  Subtract2/1 -> Transfer Fcn/1
  PWM Generator (DC-DC)1/1 -> Display2/1, Mosfet1/1
  Transfer Fcn/1 -> Gain/1  "BUCK_Ref"
  Gain/1 -> Subtract3/2, Display1/1
  Transfer Fcn1/1 -> Gain1/1, PWM Generator (DC-DC)/1
  Gain1/1 -> Subtract3/1
  Subtract3/1 -> PWM Generator (DC-DC)1/1, Display4/1
  connections:
  Diode1/LConn1 -- Series RLC Branch3/RConn1 -- Voltage Measurement1/LConn2 -- Series RLC Branch5/RConn1
  Series RLC Branch4/LConn1 -- Voltage Measurement/LConn1 -- Current Measurement2/RConn1 -- Series RLC Branch2/LConn1
  Series RLC Branch5/LConn1 -- Voltage Measurement1/LConn1 -- DC Voltage Source/LConn1 -- Voltage Measurement2/LConn2 -- Current Measurement5/RConn1 -- Diode/LConn1 -- Series RLC Branch3/LConn1 -- Series RLC Branch2/RConn1 -- Voltage Measurement/LConn2 -- Series RLC Branch4/RConn1
  Current Measurement1/LConn1 -- Series RLC Branch1/RConn1 -- Current Measurement4/LConn1
  Series RLC Branch/LConn1 -- Current Measurement/RConn1 -- Current Measurement3/LConn1
  Voltage Measurement2/LConn1 -- Mosfet/LConn1 -- DC Voltage Source/RConn1
  Diode1/RConn1 -- Current Measurement1/RConn1
  Current Measurement2/LConn1 -- Series RLC Branch/RConn1
  Current Measurement5/LConn1 -- Series RLC Branch1/LConn1
  Mosfet/RConn1 -- Mosfet1/LConn1 -- Current Measurement3/RConn1
  Current Measurement4/RConn1 -- Mosfet1/RConn1
  Current Measurement/LConn1 -- Diode/RConn1

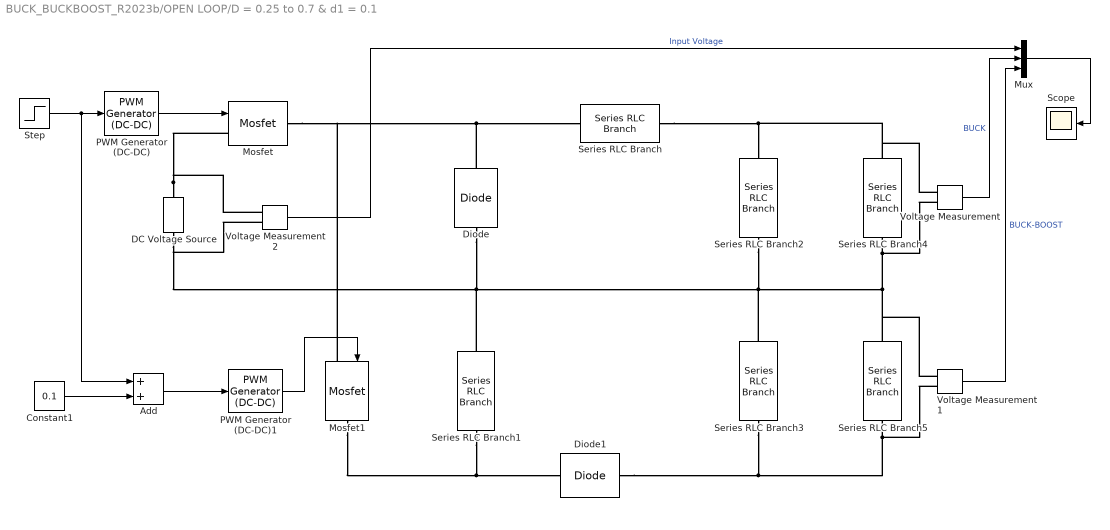
== system BUCK_BUCKBOOST_R2023b/OPEN LOOP/D = 0.25 to 0.7 & d1 = 0.1 ==
  Add : Sum
  Constant1 : Constant  Value=0.1
  DC Voltage Source : spsDCVoltageSourceLib/DC Voltage Source  Amplitude=48  Measurements=None
  Diode : spsDiodeLib/Diode  Ron=0.001  Lon=0  Vf=0.8  IC=0  UseSnubber=0  Rs=500  Cs=250e-9  Measurements=off
  Diode1 : spsDiodeLib/Diode  Ron=0.001  Lon=0  Vf=0.8  IC=0  UseSnubber=0  Rs=500  Cs=250e-9  Measurements=off
  Mosfet : spsMosfetLib/Mosfet  Ron=0.1  Lon=0  Rd=0.01  Vfd=0  IC=0  Rs=1e5  Cs=inf  Measurements=off
  Mosfet1 : spsMosfetLib/Mosfet  Ron=0.1  Lon=0  Rd=0.01  Vfd=0  IC=0  Rs=1e5  Cs=inf  Measurements=off
  Mux : Mux  Inputs=3
  PWM Generator (DC-DC) : spsPWMGeneratorDCDCLib/PWM Generator (DC-DC)  Fsw=50000  Ts=0
  PWM Generator (DC-DC)1 : spsPWMGeneratorDCDCLib/PWM Generator (DC-DC)  Fsw=50000  Ts=0
  Scope : Scope
  Series RLC Branch : spsSeriesRLCBranchLib/Series RLC Branch  LConnTagsString=__new0  RConnTagsString=__new0  BranchType=L  Resistance=1  Inductance=2e-3  SetiL0=off  InitialCurrent=0  Capacitance=1e-6  Setx0=off  InitialVoltage=0  Measurements=None
  Series RLC Branch1 : spsSeriesRLCBranchLib/Series RLC Branch  LConnTagsString=__new0  RConnTagsString=__new0  BranchType=L  Resistance=1  Inductance=600e-6  SetiL0=off  InitialCurrent=0  Capacitance=1e-6  Setx0=off  InitialVoltage=0  Measurements=None
  Series RLC Branch2 : spsSeriesRLCBranchLib/Series RLC Branch  LConnTagsString=__new0  RConnTagsString=__new0  BranchType=C  Resistance=1  Inductance=1e-3  SetiL0=off  InitialCurrent=0  Capacitance=100e-6  Setx0=off  InitialVoltage=0  Measurements=None
  Series RLC Branch3 : spsSeriesRLCBranchLib/Series RLC Branch  LConnTagsString=__new0  RConnTagsString=__new0  BranchType=C  Resistance=1  Inductance=1e-3  SetiL0=off  InitialCurrent=0  Capacitance=100e-6  Setx0=off  InitialVoltage=0  Measurements=None
  Series RLC Branch4 : spsSeriesRLCBranchLib/Series RLC Branch  LConnTagsString=__new0  RConnTagsString=__new0  BranchType=R  Resistance=100  Inductance=1e-3  SetiL0=off  InitialCurrent=0  Capacitance=1e-6  Setx0=off  InitialVoltage=0  Measurements=None
  Series RLC Branch5 : spsSeriesRLCBranchLib/Series RLC Branch  LConnTagsString=__new0  RConnTagsString=__new0  BranchType=R  Resistance=100  Inductance=1e-3  SetiL0=off  InitialCurrent=0  Capacitance=1e-6  Setx0=off  InitialVoltage=0  Measurements=None
  Step : Step  Time=0.5  Before=0.25  After=0.7  SampleTime=0
  Voltage Measurement : spsVoltageMeasurementLib/Voltage Measurement  PhasorSimulation=off  OutputType=Complex  PSBequivalent=0
  Voltage Measurement1 : spsVoltageMeasurementLib/Voltage Measurement  PhasorSimulation=off  OutputType=Complex  PSBequivalent=0
  Voltage Measurement2 : spsVoltageMeasurementLib/Voltage Measurement  PhasorSimulation=off  OutputType=Complex  PSBequivalent=0
  wires:
  Step/1 -> Add/1, PWM Generator (DC-DC)/1
  Voltage Measurement2/1 -> Mux/1  "Input Voltage"
  Add/1 -> PWM Generator (DC-DC)1/1
  Mux/1 -> Scope/1
  PWM Generator (DC-DC)/1 -> Mosfet/1
  PWM Generator (DC-DC)1/1 -> Mosfet1/1
  Voltage Measurement1/1 -> Mux/3  "BUCK-BOOST"
  Voltage Measurement/1 -> Mux/2  "BUCK"
  Constant1/1 -> Add/2
  connections:
  Series RLC Branch3/RConn1 -- Diode1/LConn1 -- Voltage Measurement1/LConn2 -- Series RLC Branch5/RConn1
  Series RLC Branch/RConn1 -- Series RLC Branch2/LConn1 -- Series RLC Branch4/LConn1 -- Voltage Measurement/LConn1
  Series RLC Branch1/LConn1 -- Diode/LConn1 -- DC Voltage Source/LConn1 -- Voltage Measurement2/LConn2 -- Series RLC Branch3/LConn1 -- Series RLC Branch2/RConn1 -- Voltage Measurement1/LConn1 -- Series RLC Branch5/LConn1 -- Voltage Measurement/LConn2 -- Series RLC Branch4/RConn1
  Series RLC Branch1/RConn1 -- Mosfet1/RConn1 -- Diode1/RConn1
  Diode/RConn1 -- Series RLC Branch/LConn1 -- Mosfet/RConn1 -- Mosfet1/LConn1
  DC Voltage Source/RConn1 -- Mosfet/LConn1 -- Voltage Measurement2/LConn1

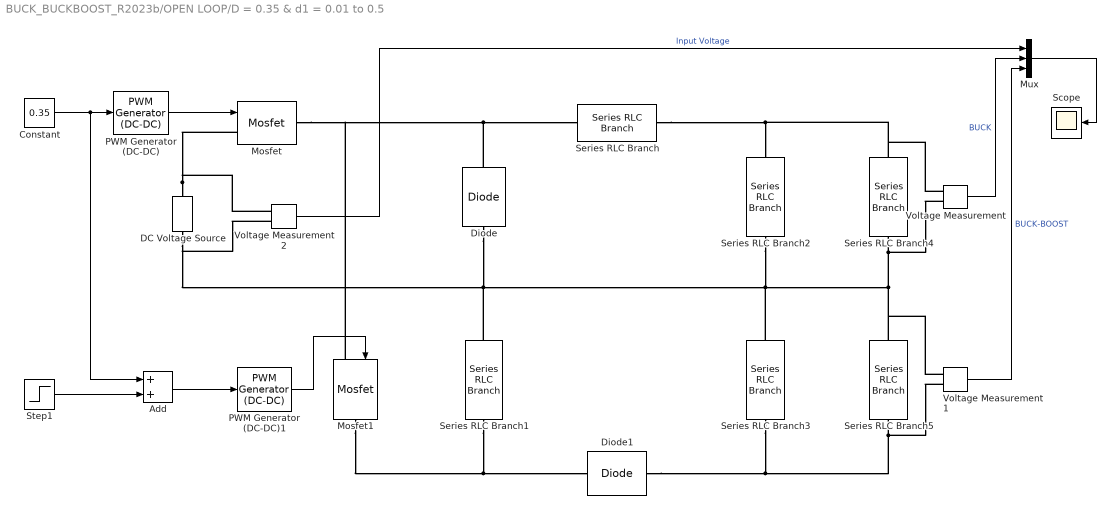
== system BUCK_BUCKBOOST_R2023b/OPEN LOOP/D = 0.35 & d1 = 0.01 to 0.5 ==
  Add : Sum
  Constant : Constant  Value=0.35
  DC Voltage Source : spsDCVoltageSourceLib/DC Voltage Source  Amplitude=48  Measurements=None
  Diode : spsDiodeLib/Diode  Ron=0.001  Lon=0  Vf=0.8  IC=0  UseSnubber=0  Rs=500  Cs=250e-9  Measurements=off
  Diode1 : spsDiodeLib/Diode  Ron=0.001  Lon=0  Vf=0.8  IC=0  UseSnubber=0  Rs=500  Cs=250e-9  Measurements=off
  Mosfet : spsMosfetLib/Mosfet  Ron=0.1  Lon=0  Rd=0.01  Vfd=0  IC=0  Rs=1e5  Cs=inf  Measurements=off
  Mosfet1 : spsMosfetLib/Mosfet  Ron=0.1  Lon=0  Rd=0.01  Vfd=0  IC=0  Rs=1e5  Cs=inf  Measurements=off
  Mux : Mux  Inputs=3
  PWM Generator (DC-DC) : spsPWMGeneratorDCDCLib/PWM Generator (DC-DC)  Fsw=50000  Ts=0
  PWM Generator (DC-DC)1 : spsPWMGeneratorDCDCLib/PWM Generator (DC-DC)  Fsw=50000  Ts=0
  Scope : Scope
  Series RLC Branch : spsSeriesRLCBranchLib/Series RLC Branch  LConnTagsString=__new0  RConnTagsString=__new0  BranchType=L  Resistance=1  Inductance=2e-3  SetiL0=off  InitialCurrent=0  Capacitance=1e-6  Setx0=off  InitialVoltage=0  Measurements=None
  Series RLC Branch1 : spsSeriesRLCBranchLib/Series RLC Branch  LConnTagsString=__new0  RConnTagsString=__new0  BranchType=L  Resistance=1  Inductance=600e-6  SetiL0=off  InitialCurrent=0  Capacitance=1e-6  Setx0=off  InitialVoltage=0  Measurements=None
  Series RLC Branch2 : spsSeriesRLCBranchLib/Series RLC Branch  LConnTagsString=__new0  RConnTagsString=__new0  BranchType=C  Resistance=1  Inductance=1e-3  SetiL0=off  InitialCurrent=0  Capacitance=100e-6  Setx0=off  InitialVoltage=0  Measurements=None
  Series RLC Branch3 : spsSeriesRLCBranchLib/Series RLC Branch  LConnTagsString=__new0  RConnTagsString=__new0  BranchType=C  Resistance=1  Inductance=1e-3  SetiL0=off  InitialCurrent=0  Capacitance=100e-6  Setx0=off  InitialVoltage=0  Measurements=None
  Series RLC Branch4 : spsSeriesRLCBranchLib/Series RLC Branch  LConnTagsString=__new0  RConnTagsString=__new0  BranchType=R  Resistance=100  Inductance=1e-3  SetiL0=off  InitialCurrent=0  Capacitance=1e-6  Setx0=off  InitialVoltage=0  Measurements=None
  Series RLC Branch5 : spsSeriesRLCBranchLib/Series RLC Branch  LConnTagsString=__new0  RConnTagsString=__new0  BranchType=R  Resistance=100  Inductance=1e-3  SetiL0=off  InitialCurrent=0  Capacitance=1e-6  Setx0=off  InitialVoltage=0  Measurements=None
  Step1 : Step  Time=0.5  Before=0.01  After=0.5  SampleTime=0
  Voltage Measurement : spsVoltageMeasurementLib/Voltage Measurement  PhasorSimulation=off  OutputType=Complex  PSBequivalent=0
  Voltage Measurement1 : spsVoltageMeasurementLib/Voltage Measurement  PhasorSimulation=off  OutputType=Complex  PSBequivalent=0
  Voltage Measurement2 : spsVoltageMeasurementLib/Voltage Measurement  PhasorSimulation=off  OutputType=Complex  PSBequivalent=0
  wires:
  Constant/1 -> Add/1, PWM Generator (DC-DC)/1
  Voltage Measurement2/1 -> Mux/1  "Input Voltage"
  Add/1 -> PWM Generator (DC-DC)1/1
  Mux/1 -> Scope/1
  PWM Generator (DC-DC)/1 -> Mosfet/1
  PWM Generator (DC-DC)1/1 -> Mosfet1/1
  Voltage Measurement1/1 -> Mux/3  "BUCK-BOOST"
  Voltage Measurement/1 -> Mux/2  "BUCK"
  Step1/1 -> Add/2
  connections:
  Series RLC Branch3/RConn1 -- Diode1/LConn1 -- Series RLC Branch5/RConn1 -- Voltage Measurement1/LConn2
  Series RLC Branch/RConn1 -- Series RLC Branch2/LConn1 -- Series RLC Branch4/LConn1 -- Voltage Measurement/LConn1
  Series RLC Branch1/LConn1 -- Diode/LConn1 -- Series RLC Branch3/LConn1 -- Series RLC Branch2/RConn1 -- Voltage Measurement1/LConn1 -- Series RLC Branch5/LConn1 -- Voltage Measurement/LConn2 -- Series RLC Branch4/RConn1 -- DC Voltage Source/LConn1 -- Voltage Measurement2/LConn2
  Series RLC Branch1/RConn1 -- Mosfet1/RConn1 -- Diode1/RConn1
  Diode/RConn1 -- Series RLC Branch/LConn1 -- Mosfet/RConn1 -- Mosfet1/LConn1
  DC Voltage Source/RConn1 -- Mosfet/LConn1 -- Voltage Measurement2/LConn1

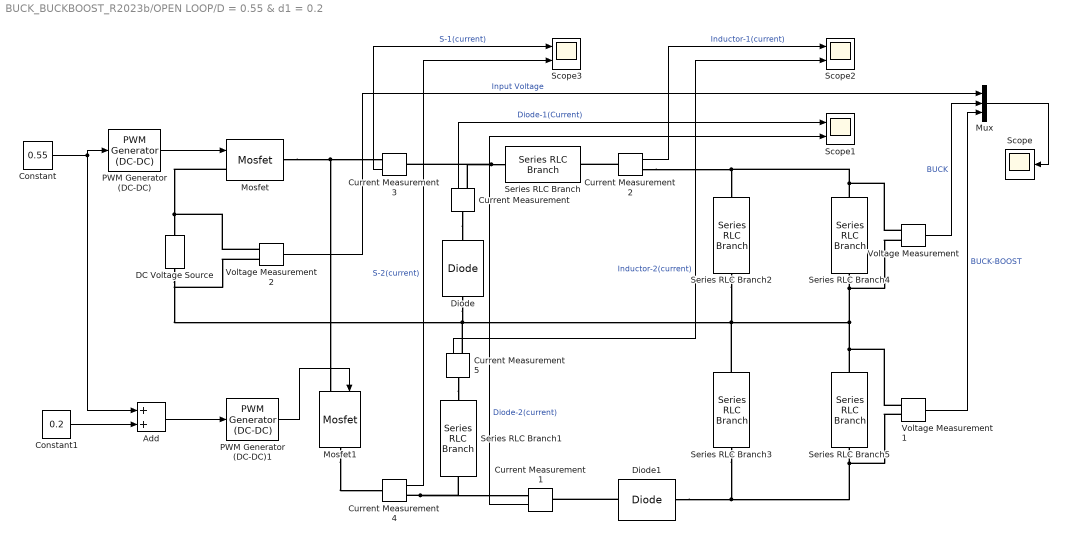
== system BUCK_BUCKBOOST_R2023b/OPEN LOOP/D = 0.55 & d1 = 0.2 ==
  Add : Sum
  Constant : Constant  Value=0.55
  Constant1 : Constant  Value=0.2
  Current Measurement{,1..5} (6 alike) : spsCurrentMeasurementLib/Current Measurement  PhasorSimulation=off  OutputType=Complex  PSBequivalent=0
  DC Voltage Source : spsDCVoltageSourceLib/DC Voltage Source  Amplitude=48  Measurements=None
  Diode : spsDiodeLib/Diode  Ron=0.001  Lon=0  Vf=0.8  IC=0  UseSnubber=0  Rs=500  Cs=250e-9  Measurements=off
  Diode1 : spsDiodeLib/Diode  Ron=0.001  Lon=0  Vf=0.8  IC=0  UseSnubber=0  Rs=500  Cs=250e-9  Measurements=off
  Mosfet : spsMosfetLib/Mosfet  Ron=0.1  Lon=0  Rd=0.01  Vfd=0  IC=0  Rs=1e5  Cs=inf  Measurements=off
  Mosfet1 : spsMosfetLib/Mosfet  Ron=0.1  Lon=0  Rd=0.01  Vfd=0  IC=0  Rs=1e5  Cs=inf  Measurements=off
  Mux : Mux  Inputs=3
  PWM Generator (DC-DC) : spsPWMGeneratorDCDCLib/PWM Generator (DC-DC)  Fsw=50000  Ts=0
  PWM Generator (DC-DC)1 : spsPWMGeneratorDCDCLib/PWM Generator (DC-DC)  Fsw=50000  Ts=0
  Scope : Scope
  Scope1 : Scope  NumInputPorts=2
  Scope2 : Scope  NumInputPorts=2
  Scope3 : Scope  NumInputPorts=2
  Series RLC Branch : spsSeriesRLCBranchLib/Series RLC Branch  LConnTagsString=__new0  RConnTagsString=__new0  BranchType=L  Resistance=1  Inductance=2e-3  SetiL0=off  InitialCurrent=0  Capacitance=1e-6  Setx0=off  InitialVoltage=0  Measurements=None
  Series RLC Branch1 : spsSeriesRLCBranchLib/Series RLC Branch  LConnTagsString=__new0  RConnTagsString=__new0  BranchType=L  Resistance=1  Inductance=600e-6  SetiL0=off  InitialCurrent=0  Capacitance=1e-6  Setx0=off  InitialVoltage=0  Measurements=None
  Series RLC Branch2 : spsSeriesRLCBranchLib/Series RLC Branch  LConnTagsString=__new0  RConnTagsString=__new0  BranchType=C  Resistance=1  Inductance=1e-3  SetiL0=off  InitialCurrent=0  Capacitance=100e-6  Setx0=off  InitialVoltage=0  Measurements=None
  Series RLC Branch3 : spsSeriesRLCBranchLib/Series RLC Branch  LConnTagsString=__new0  RConnTagsString=__new0  BranchType=C  Resistance=1  Inductance=1e-3  SetiL0=off  InitialCurrent=0  Capacitance=100e-6  Setx0=off  InitialVoltage=0  Measurements=None
  Series RLC Branch4 : spsSeriesRLCBranchLib/Series RLC Branch  LConnTagsString=__new0  RConnTagsString=__new0  BranchType=R  Resistance=100  Inductance=1e-3  SetiL0=off  InitialCurrent=0  Capacitance=1e-6  Setx0=off  InitialVoltage=0  Measurements=None
  Series RLC Branch5 : spsSeriesRLCBranchLib/Series RLC Branch  LConnTagsString=__new0  RConnTagsString=__new0  BranchType=R  Resistance=100  Inductance=1e-3  SetiL0=off  InitialCurrent=0  Capacitance=1e-6  Setx0=off  InitialVoltage=0  Measurements=None
  Voltage Measurement : spsVoltageMeasurementLib/Voltage Measurement  PhasorSimulation=off  OutputType=Complex  PSBequivalent=0
  Voltage Measurement1 : spsVoltageMeasurementLib/Voltage Measurement  PhasorSimulation=off  OutputType=Complex  PSBequivalent=0
  Voltage Measurement2 : spsVoltageMeasurementLib/Voltage Measurement  PhasorSimulation=off  OutputType=Complex  PSBequivalent=0
  wires:
  Constant/1 -> Add/1, PWM Generator (DC-DC)/1
  Voltage Measurement2/1 -> Mux/1  "Input Voltage"
  Add/1 -> PWM Generator (DC-DC)1/1
  Mux/1 -> Scope/1
  PWM Generator (DC-DC)/1 -> Mosfet/1
  PWM Generator (DC-DC)1/1 -> Mosfet1/1
  Voltage Measurement1/1 -> Mux/3  "BUCK-BOOST"
  Voltage Measurement/1 -> Mux/2  "BUCK"
  Constant1/1 -> Add/2
  Current Measurement/1 -> Scope1/1  "Diode-1(Current)"
  Current Measurement1/1 -> Scope1/2  "Diode-2(current)"
  Current Measurement2/1 -> Scope2/1  "Inductor-1(current)"
  Current Measurement5/1 -> Scope2/2  "Inductor-2(current)"
  Current Measurement3/1 -> Scope3/1  "S-1(current)"
  Current Measurement4/1 -> Scope3/2  "S-2(current)"
  connections:
  Diode1/LConn1 -- Series RLC Branch3/RConn1 -- Voltage Measurement1/LConn2 -- Series RLC Branch5/RConn1
  Series RLC Branch4/LConn1 -- Voltage Measurement/LConn1 -- Current Measurement2/RConn1 -- Series RLC Branch2/LConn1
  Series RLC Branch5/LConn1 -- Current Measurement5/RConn1 -- Voltage Measurement2/LConn2 -- DC Voltage Source/LConn1 -- Diode/LConn1 -- Series RLC Branch3/LConn1 -- Series RLC Branch2/RConn1 -- Voltage Measurement/LConn2 -- Series RLC Branch4/RConn1 -- Voltage Measurement1/LConn1
  Current Measurement4/RConn1 -- Series RLC Branch1/RConn1 -- Current Measurement1/RConn1
  Series RLC Branch/LConn1 -- Current Measurement/RConn1 -- Current Measurement3/LConn1
  Mosfet/LConn1 -- Voltage Measurement2/LConn1 -- DC Voltage Source/RConn1
  Diode1/RConn1 -- Current Measurement1/LConn1
  Current Measurement2/LConn1 -- Series RLC Branch/RConn1
  Current Measurement5/LConn1 -- Series RLC Branch1/LConn1
  Mosfet/RConn1 -- Mosfet1/LConn1 -- Current Measurement3/RConn1
  Mosfet1/RConn1 -- Current Measurement4/LConn1
  Current Measurement/LConn1 -- Diode/RConn1
